simulink model "blordem1_2011a"  (Simulink 7.7)
settings: Solver=ode45  SolverMode=SingleTasking  StartTime=0.0  StopTime=20  RelTol=1e-3
settings Model: Creator=T-Gamer  LastModifiedBy=Matheus Souza  CovMetricSettings=dwe  CovHtmlReporting=off  covSaveCumulativeToWorkspaceVar=off  CovSaveSingleToWorkspaceVar=off  CovExternalEMLEnable=on
settings DataIOCC: LimitDataPoints=off  SaveFormat=StructureWithTime  SignalLoggingSaveFormat=Dataset  SaveOutput=off  SaveTime=off
settings OptimizationCC: ExpressionDepthLimit=128
settings DebuggingCC: UnderspecifiedInitializationDetection=Simplified  MergeDetectMultiDrivingBlocksExec=error  SolverPrmCheckMsg=none  FcnCallInpInsideContextMsg=Enable All  StateNameClashWarn=none  SFUnexpectedBacktrackingDiag=error  SFNoUnconditionalDefaultTransitionDiag=error
settings HardwareCC: ProdBitPerPointer=64  ProdLargestAtomicFloat=Float  ProdIntDivRoundTo=Zero  ProdEndianess=LittleEndian  ProdHWDeviceType=Specified
settings CodeAppCC: CustomSymbolStrType=$N$R$M_T
settings GRTTargetCC: TargetFunctionLibrary=C99 (ISO)  GeneratePreprocessorConditionals=Use local settings

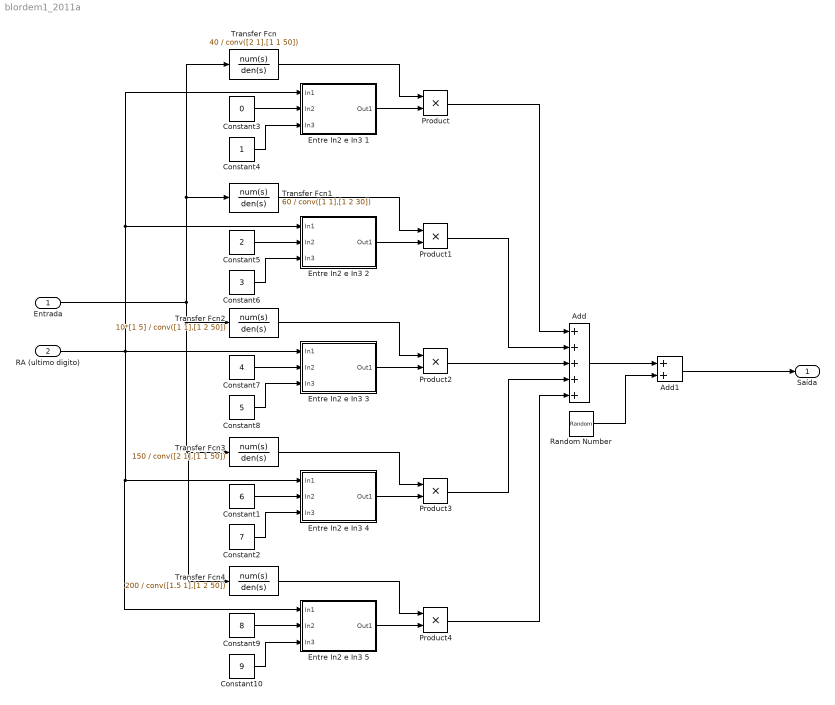
== system blordem1_2011a ==
  Entrada : Inport  OutDataTypeStr=double  PortDimensions=1  SampleTime=0
  "RA (ultimo digito) " : Inport  Port=2  OutDataTypeStr=double  PortDimensions=1  SampleTime=0
  Add : Sum  Inputs=+++++
  Add1 : Sum
  Constant1 : Constant  Value=6
  Constant10 : Constant  Value=9
  Constant2 : Constant  Value=7
  Constant3 : Constant  Value=0
  Constant4 : Constant
  Constant5 : Constant  Value=2
  Constant6 : Constant  Value=3
  Constant7 : Constant  Value=4
  Constant8 : Constant  Value=5
  Constant9 : Constant  Value=8
  Entre In2 e In3 1 : Subsystem
  Entre In2 e In3 2 : Subsystem
  Entre In2 e In3 3 : Subsystem
  Entre In2 e In3 4 : Subsystem
  Entre In2 e In3 5 : Subsystem
  Product{,1..4} (5 alike) : Product
  Random Number : RandomNumber  Variance=1e-4  SampleTime=.01
  Transfer Fcn : TransferFcn  Numerator=40  Denominator=conv([2 1],[1 1 50])
  Transfer Fcn1 : TransferFcn  Numerator=60  Denominator=conv([1 1],[1 2 30])
  Transfer Fcn2 : TransferFcn  Numerator=10*[1 5]  Denominator=conv([1 1],[1 2 50])
  Transfer Fcn3 : TransferFcn  Numerator=150  Denominator=conv([2 1],[1 1 50])
  Transfer Fcn4 : TransferFcn  Numerator=200  Denominator=conv([1.5 1],[1 2 50])
  Saída : Outport  OutDataTypeStr=double  PortDimensions=1  SampleTime=0
  wires:
  Entrada/1 -> Transfer Fcn/1, Transfer Fcn1/1, Transfer Fcn2/1, Transfer Fcn3/1, Transfer Fcn4/1
  Add/1 -> Add1/1
  Entre In2 e In3 1/1(Out1) -> Product/2
  Constant3/1 -> Entre In2 e In3 1/2(In2)
  Constant4/1 -> Entre In2 e In3 1/3(In3)
  Random Number/1 -> Add1/2
  Constant8/1 -> Entre In2 e In3 3/3(In3)
  Transfer Fcn3/1 -> Product3/1
  Constant6/1 -> Entre In2 e In3 2/3(In3)
  Product1/1 -> Add/2
  Transfer Fcn/1 -> Product/1
  Constant5/1 -> Entre In2 e In3 2/2(In2)
  Entre In2 e In3 4/1(Out1) -> Product3/2
  Constant2/1 -> Entre In2 e In3 4/3(In3)
  Constant1/1 -> Entre In2 e In3 4/2(In2)
  Product4/1 -> Add/5
  Constant10/1 -> Entre In2 e In3 5/3(In3)
  Constant7/1 -> Entre In2 e In3 3/2(In2)
  Transfer Fcn2/1 -> Product2/1
  Entre In2 e In3 3/1(Out1) -> Product2/2
  Product/1 -> Add/1
  "RA (ultimo digito) "/1 -> Entre In2 e In3 1/1(In1), Entre In2 e In3 2/1(In1), Entre In2 e In3 3/1(In1), Entre In2 e In3 4/1(In1), Entre In2 e In3 5/1(In1)
  Transfer Fcn1/1 -> Product1/1
  Product3/1 -> Add/4
  Entre In2 e In3 2/1(Out1) -> Product1/2
  Constant9/1 -> Entre In2 e In3 5/2(In2)
  Entre In2 e In3 5/1(Out1) -> Product4/2
  Transfer Fcn4/1 -> Product4/1
  Product2/1 -> Add/3
  Add1/1 -> Saída/1

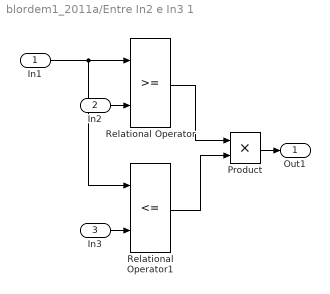
== system blordem1_2011a/Entre In2 e In3 1 ==
  In1 : Inport
  In2 : Inport  Port=2
  In3 : Inport  Port=3
  Product : Product
  Relational Operator : RelationalOperator  OutDataTypeStr=boolean
  Relational Operator1 : RelationalOperator  Operator=<=  OutDataTypeStr=boolean
  Out1 : Outport
  wires:
  In1/1 -> Relational Operator1/1, Relational Operator/1
  Relational Operator1/1 -> Product/2
  Relational Operator/1 -> Product/1
  Product/1 -> Out1/1
  In3/1 -> Relational Operator1/2
  In2/1 -> Relational Operator/2

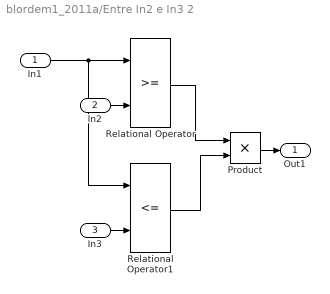
== system blordem1_2011a/Entre In2 e In3 2 ==
  In1 : Inport
  In2 : Inport  Port=2
  In3 : Inport  Port=3
  Product : Product
  Relational Operator : RelationalOperator  OutDataTypeStr=boolean
  Relational Operator1 : RelationalOperator  Operator=<=  OutDataTypeStr=boolean
  Out1 : Outport
  wires:
  In2/1 -> Relational Operator/2
  In3/1 -> Relational Operator1/2
  Product/1 -> Out1/1
  Relational Operator/1 -> Product/1
  Relational Operator1/1 -> Product/2
  In1/1 -> Relational Operator/1, Relational Operator1/1

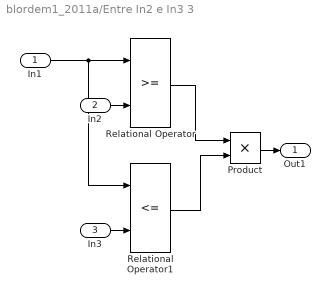
== system blordem1_2011a/Entre In2 e In3 3 ==
  In1 : Inport
  In2 : Inport  Port=2
  In3 : Inport  Port=3
  Product : Product
  Relational Operator : RelationalOperator  OutDataTypeStr=boolean
  Relational Operator1 : RelationalOperator  Operator=<=  OutDataTypeStr=boolean
  Out1 : Outport
  wires:
  In1/1 -> Relational Operator1/1, Relational Operator/1
  Relational Operator1/1 -> Product/2
  Relational Operator/1 -> Product/1
  Product/1 -> Out1/1
  In3/1 -> Relational Operator1/2
  In2/1 -> Relational Operator/2

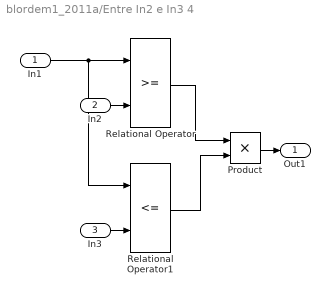
== system blordem1_2011a/Entre In2 e In3 4 ==
  In1 : Inport
  In2 : Inport  Port=2
  In3 : Inport  Port=3
  Product : Product
  Relational Operator : RelationalOperator  OutDataTypeStr=boolean
  Relational Operator1 : RelationalOperator  Operator=<=  OutDataTypeStr=boolean
  Out1 : Outport
  wires:
  In2/1 -> Relational Operator/2
  In3/1 -> Relational Operator1/2
  Product/1 -> Out1/1
  Relational Operator/1 -> Product/1
  Relational Operator1/1 -> Product/2
  In1/1 -> Relational Operator/1, Relational Operator1/1

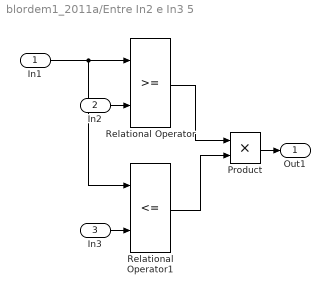
== system blordem1_2011a/Entre In2 e In3 5 ==
  In1 : Inport
  In2 : Inport  Port=2
  In3 : Inport  Port=3
  Product : Product
  Relational Operator : RelationalOperator  OutDataTypeStr=boolean
  Relational Operator1 : RelationalOperator  Operator=<=  OutDataTypeStr=boolean
  Out1 : Outport
  wires:
  In1/1 -> Relational Operator1/1, Relational Operator/1
  Relational Operator1/1 -> Product/2
  Relational Operator/1 -> Product/1
  Product/1 -> Out1/1
  In3/1 -> Relational Operator1/2
  In2/1 -> Relational Operator/2
